simulink model "FreqSweep"  (Simulink 7.6)
settings: Solver=FixedStepDiscrete  SolverMode=SingleTasking  StartTime=0.0  StopTime=137*20*8*4  FixedStep=1  RelTol=1e-3
PreLoadFcn:
  | close all
  | clear all
  | FilterOrder = 32
  | InputBitWidth = 8
  | LowPassFreqBand = [0 0.01 0.2 1];
  | LowPassMagnBand = [1 0.9 0.0001 0.0001];
  | 
  | FlCoef = firls(FilterOrder,LowPassFreqBand,LowPassMagnBand);
  | 
  | CoefBitWidth = InputBitWidth + ceil(log2((max(abs(FlCoef))/min(abs(FlCoef)))))
  | 
  | ScalingFactor = (2^(CoefBitWidth-1))-1;
  | FpCoef = fix(ScalingFactor * FlCoef);
  | %plot(FpCoef,'o');
  | %title('Fixed-point scaled coefficient value');
  | ImpulseData = zeros(1,1000);
  | ImpulseData(1) = 100;
  | h = conv(ImpulseData,FpCoef);
  | %fftplot(h);
  | %title('FIR Frequency response');
  | FirSamplingPeriod=1;
  | 
  | cordic_precision=20;
  | ScalingFactor = (2^(cordic_precision-1))-1;
  | K=1.0;
  | for i=1:cordic_precision
  |   cordic_atan_table(i) = round(atan(K)*ScalingFactor);
  |   K=0.5*K;
  | end;
  | %disp(['cordic_precision =' num2str(cordic_precision)]);
  | %disp(['cordic_atan_table =' num2str(cordic_atan_table)]);
InitFcn:
  | %% DSPBuilder Start
  | alt_dspbuilder_update_model(bdroot)
  | %% DSPBuilder End
libraries: allblocks_alteradspbuilder2 x97, simulink x1
settings Model: Creator=akarapet  LastModifiedBy=akarapet
settings DataIOCC: SignalLoggingName=sigsOut
settings OptimizationCC: InlineInvariantSignals=on  InitFltsAndDblsToZero=on
settings DebuggingCC: SaveWithParameterizedLinksMsg=none  SignalResolutionControl=TryResolveAllWithWarning  SolverPrmCheckMsg=none  MultiTaskDSMMsg=warning  MultiTaskCondExecSysMsg=none  StrictBusMsg=None
settings HardwareCC: TargetUnknown=on
settings RTWCC: IncludeERTFirstTime=on
settings GRTTargetCC: TargetFcnLib=ansi_tfl_tmw.mat

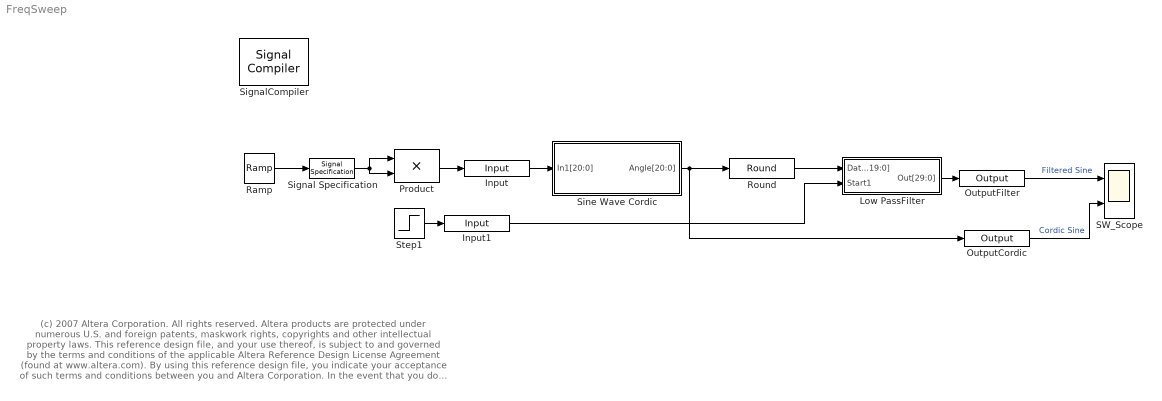
== system FreqSweep ==
  note: (c) 2007 Altera Corporation. All rights reserved.  Altera products are protected under numerous U.S. and foreign patents, maskwork rights, copyrights and other intellectual property laws.
      | This reference design file, and your use thereof, is subject to and governed by the terms and conditions of the applicable Altera Reference Design License Agreement (found at www.altera.com).
      | By using this reference design file, you indicate your acceptance of such terms and conditions between you and Altera Corporation.
      | In the event that you do not agree with such terms and conditions, you may not use the reference design file and please promptly destroy any copies you have made.
      | This reference design file being provided on an "as-is" basis and as an accommodation and therefore all warranties, representations or guarantees of any kind (whether express, implied or statutory)
      | including, without limitation, warranties of merchantability, non-infringement, or fitness for a particular purpose, are specifically disclaimed.
      | By making this reference design file available, Altera expressly does not recommend, suggest or require that this reference design file be used in combination with any other product not provided by Altera
  Input : allblocks_alteradspbuilder2/Input  iofile=/data/akarapet/qshell_linux64_test/p4/dsp_builder/dsp_builder2/Documentation/DesignExamples/Tutorials/HIL/FreqSweep/tb_FreqSweep/FreqSweep_Input.salt  BusType=Unsigned Integer  bwl=21  bwr=0  SpecifyClock=off  PORTTYPE=Input  externalType=Inferred  allowFloatingPointOverride=on  logOutputs=off
  Input1 : allblocks_alteradspbuilder2/Input  iofile=/data/akarapet/qshell_linux64_test/p4/dsp_builder/dsp_builder2/Documentation/DesignExamples/Tutorials/HIL/FreqSweep/tb_FreqSweep/FreqSweep_Input1.salt  BusType=Single Bit  bwl=1  bwr=0  SpecifyClock=off  PORTTYPE=Input  externalType=Inferred  allowFloatingPointOverride=on  logOutputs=off
  Low PassFilter : Subsystem  AncestorBlock=ALTELINK/AltLab/HDL SubSystem
      mask Type: SubSystem AlteraBlockSet
  OutputCordic : allblocks_alteradspbuilder2/Output  iofile=/data/akarapet/qshell_linux64_test/p4/dsp_builder/dsp_builder2/Documentation/DesignExamples/Tutorials/HIL/FreqSweep/tb_FreqSweep/FreqSweep_OutputCordic.capture  BusType=Signed Integer  bwl=21  bwr=0  externalType=Inferred  PORTTYPE=Output  allowFloatingPointOverride=on  logOutputs=off
  OutputFilter : allblocks_alteradspbuilder2/Output  iofile=/data/akarapet/qshell_linux64_test/p4/dsp_builder/dsp_builder2/Documentation/DesignExamples/Tutorials/HIL/FreqSweep/tb_FreqSweep/FreqSweep_OutputFilter.capture  BusType=Signed Integer  bwl=30  bwr=0  externalType=Inferred  PORTTYPE=Output  allowFloatingPointOverride=on  logOutputs=off
  Product : Product  SaturateOnIntegerOverflow=on  OutDataTypeStr=Inherit: Same as first input
  Ramp : simulink/Sources/Ramp  SystemSampleTime=-1  slope=.01  start=0  X0=0
  Round : allblocks_alteradspbuilder2/Round  BusType=Signed Integer  bwl=21  bwr=0  bitsToRemove=1  roundMode=ROUND_UP_SYM  userRoundMode=Round Away From Zero  pipeline=on  pipeline_display=1  use_ena=off  use_aclr=off
  SW_Scope : Scope  NumInputPorts=2
      settings: YMin=-1.1e+006~-550000  YMax=1.1e+006~550000  Decimation=20
  Signal Specification : SignalSpecification  SampleTime=1
  SignalCompiler : allblocks_alteradspbuilder2/Signal Compiler  DeviceFamily=Cyclone III  DeviceName=EP3C120F780C7  EnableSignalTap=off  SignalTapDepth=128  UseBoardBlock=off  StpUseDefaultClock=on  StpClock=Clock  ExportDir=/data/akarapet/qshell_linux64_test/p4/dsp_builder/dsp_builder2/Documentation/DesignExamples/Tutorials/HIL/FreqSweep/.
  Sine Wave Cordic : Subsystem
      mask Type: SubSystem AlteraBlockSet
  Step1 : Step  SampleTime=1
  wires:
  Ramp/1 -> Signal Specification/1
  Sine Wave Cordic/1(Angle[20:0]) -> OutputCordic/1, Round/1
  Input1/1 -> Low PassFilter/2(Start1)
  Step1/1 -> Input1/1
  Round/1 -> Low PassFilter/1(DataIn[19:0])
  Product/1 -> Input/1
  Input/1 -> Sine Wave Cordic/1(In1[20:0])
  Low PassFilter/1(Out[29:0]) -> OutputFilter/1
  Signal Specification/1 -> Product/1, Product/2
  OutputFilter/1 -> SW_Scope/1  "Filtered Sine"
  OutputCordic/1 -> SW_Scope/2  "Cordic Sine"

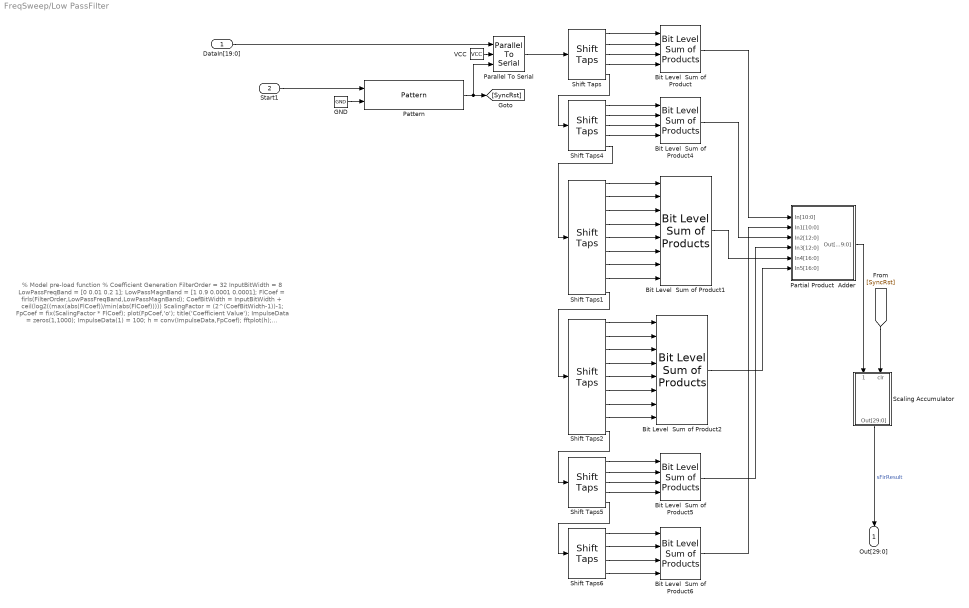
== system FreqSweep/Low PassFilter ==
  note: % Model pre-load function
      | % Coefficient Generation
      | FilterOrder = 32
      | InputBitWidth = 8
      | LowPassFreqBand = [0 0.01 0.2 1];
      | LowPassMagnBand = [1 0.9 0.0001 0.0001];
      |
      | FlCoef = firls(FilterOrder,LowPassFreqBand,LowPassMagnBand);
      |
      | CoefBitWidth = InputBitWidth + ceil(log2((max(abs(FlCoef))/min(abs(FlCoef)))))
      | ScalingFactor = (2^(CoefBitWidth-1))-1;
      |
      | FpCoef = fix(ScalingFactor * FlCoef);
      |
      | plot(FpCoef,'o');
      | title('Coefficient Value');
      | ImpulseData = zeros(1,1000);
      | ImpulseData(1) = 100;
      | h = conv(ImpulseData,FpCoef);
      | fftplot(h);
      | title('Frequency response');
      | FirSamplingPeriod=1;
  DataIn[19:0] : Inport
  Start1 : Inport  Port=2
  Bit Level  Sum of Product : allblocks_alteradspbuilder2/Bit Level Sum of Products  number_of_coefficients=4  BusType=Signed Integer  bwl=9  bwr=0  coefficients=[FpCoef(1:4)]  register_inputs=off  pipeline_display=0  use_ena=off  use_sclr=off  allowFloatingPointOverride=on  logOutputs=off  logFile=/data/akarapet/qshell_linux64_test/p4/dsp_builder/dsp_builder2/Documentation/DesignExamples/Tutorials/HIL/FreqSweep/tb_FreqSweep/FreqSweep_Low+PassFilter_Bit+Level+%0ASum+of+Product.fixedpointlog
  Bit Level  Sum of Product1 : allblocks_alteradspbuilder2/Bit Level Sum of Products  number_of_coefficients=8  BusType=Signed Integer  bwl=14  bwr=0  coefficients=[FpCoef(9:16)]  register_inputs=off  pipeline_display=0  use_ena=off  use_sclr=off  allowFloatingPointOverride=on  logOutputs=off  logFile=/data/akarapet/qshell_linux64_test/p4/dsp_builder/dsp_builder2/Documentation/DesignExamples/Tutorials/HIL/FreqSweep/tb_FreqSweep/FreqSweep_Low+PassFilter_Bit+Level+%0ASum+of+Product1.fixedpointlog
  Bit Level  Sum of Product2 : allblocks_alteradspbuilder2/Bit Level Sum of Products  number_of_coefficients=8  BusType=Signed Integer  bwl=14  bwr=0  coefficients=[FpCoef(17:24)]  register_inputs=off  pipeline_display=0  use_ena=off  use_sclr=off  allowFloatingPointOverride=on  logOutputs=off  logFile=/data/akarapet/qshell_linux64_test/p4/dsp_builder/dsp_builder2/Documentation/DesignExamples/Tutorials/HIL/FreqSweep/tb_FreqSweep/FreqSweep_Low+PassFilter_Bit+Level+%0ASum+of+Product2.fixedpointlog
  Bit Level  Sum of Product4 : allblocks_alteradspbuilder2/Bit Level Sum of Products  number_of_coefficients=4  BusType=Signed Integer  bwl=11  bwr=0  coefficients=[FpCoef(5:8)]  register_inputs=off  pipeline_display=0  use_ena=off  use_sclr=off  allowFloatingPointOverride=on  logOutputs=off  logFile=/data/akarapet/qshell_linux64_test/p4/dsp_builder/dsp_builder2/Documentation/DesignExamples/Tutorials/HIL/FreqSweep/tb_FreqSweep/FreqSweep_Low+PassFilter_Bit+Level+%0ASum+of+Product4.fixedpointlog
  Bit Level  Sum of Product5 : allblocks_alteradspbuilder2/Bit Level Sum of Products  number_of_coefficients=4  BusType=Signed Integer  bwl=11  bwr=0  coefficients=[FpCoef(25:28)]  register_inputs=off  pipeline_display=0  use_ena=off  use_sclr=off  allowFloatingPointOverride=on  logOutputs=off  logFile=/data/akarapet/qshell_linux64_test/p4/dsp_builder/dsp_builder2/Documentation/DesignExamples/Tutorials/HIL/FreqSweep/tb_FreqSweep/FreqSweep_Low+PassFilter_Bit+Level+%0ASum+of+Product5.fixedpointlog
  Bit Level  Sum of Product6 : allblocks_alteradspbuilder2/Bit Level Sum of Products  number_of_coefficients=4  BusType=Signed Integer  bwl=9  bwr=0  coefficients=[FpCoef(29:32)]  register_inputs=off  pipeline_display=0  use_ena=off  use_sclr=off  allowFloatingPointOverride=on  logOutputs=off  logFile=/data/akarapet/qshell_linux64_test/p4/dsp_builder/dsp_builder2/Documentation/DesignExamples/Tutorials/HIL/FreqSweep/tb_FreqSweep/FreqSweep_Low+PassFilter_Bit+Level+%0ASum+of+Product6.fixedpointlog
  GND : allblocks_alteradspbuilder2/GND  SpecifyClock=off
  Parallel To Serial : allblocks_alteradspbuilder2/Parallel To Serial  BusType=Signed Integer  bwl=20  bwr=0  msbfirsttext=LSB First  msbfirst=0  repeatlastbit=on  use_ena=on  use_sclr=off
  Partial Product  Adder : Subsystem  AncestorBlock=ALTELINK/AltLab/HDL SubSystem
      mask Type: SubSystem AlteraBlockSet
  Pattern : allblocks_alteradspbuilder2/Pattern  Sequence=10000000000000000000  SpecifyClock=off  use_ena=on  use_sclr=on
  Scaling Accumulator : Subsystem  AncestorBlock=ALTELINK/AltLab/HDL SubSystem
      mask Type: SubSystem AlteraBlockSet
  Shift Taps : allblocks_alteradspbuilder2/Shift Taps  number_of_taps=4  tap_distance=20  use_shiftout=on  use_ena=off  use_sclr=off  use_dedicated_circuitry=on  ram_type=AUTO  allowFloatingPointOverride=on  logOutputs=off  logFile=/data/akarapet/qshell_linux64_test/p4/dsp_builder/dsp_builder2/Documentation/DesignExamples/Tutorials/HIL/FreqSweep/tb_FreqSweep/FreqSweep_Low+PassFilter_Shift+Taps%3A%3At.fixedpointlog,/data/akarapet/qshell_linux64_test/p4/dsp_builder/dsp_builder2/Documentation/DesignExamples/Tutorials/HIL/FreqSweep/tb_FreqSweep/FreqSweep_Low+PassFilter_Shift+Taps%3A%3At.fixedpointlog,/data/akarapet/qshell_linux64_test/p4/dsp_builder/dsp_builder2/Documentation/DesignExamples/Tutorials/HIL/FreqSweep/tb_FreqSweep/FreqSweep_Low+PassFilter_Shift+Taps%3A%3At.fixedpointlog,/data/akarapet/qshell_linux64_test/p4/dsp_builder/dsp_builder2/Documentation/DesignExamples/Tutorials/HIL/FreqSweep/tb_FreqSweep/FreqSweep_Low+PassFilter_Shift+Taps%3A%3At.fixedpointlog,/data/akarapet/qshell_linux64_test/p4/dsp_builder/dsp_builder2/Documentation/DesignExamples/Tutorials/HIL/FreqSweep/tb_FreqSweep/FreqSweep_Low+PassFilter_Shift+Taps%3A%3Ashiftout.fixedpointlog,
  Shift Taps1 : allblocks_alteradspbuilder2/Shift Taps  number_of_taps=8  tap_distance=20  use_shiftout=on  use_ena=off  use_sclr=off  use_dedicated_circuitry=on  ram_type=AUTO  allowFloatingPointOverride=on  logOutputs=off  logFile=/data/akarapet/qshell_linux64_test/p4/dsp_builder/dsp_builder2/Documentation/DesignExamples/Tutorials/HIL/FreqSweep/tb_FreqSweep/FreqSweep_Low+PassFilter_Shift+Taps1%3A%3At.fixedpointlog,/data/akarapet/qshell_linux64_test/p4/dsp_builder/dsp_builder2/Documentation/DesignExamples/Tutorials/HIL/FreqSweep/tb_FreqSweep/FreqSweep_Low+PassFilter_Shift+Taps1%3A%3At.fixedpointlog,/data/akarapet/qshell_linux64_test/p4/dsp_builder/dsp_builder2/Documentation/DesignExamples/Tutorials/HIL/FreqSweep/tb_FreqSweep/FreqSweep_Low+PassFilter_Shift+Taps1%3A%3At.fixedpointlog,/data/akarapet/qshell_linux64_test/p4/dsp_builder/dsp_builder2/Documentation/DesignExamples/Tutorials/HIL/FreqSweep/tb_FreqSweep/FreqSweep_Low+PassFilter_Shift+Taps1%3A%3At.fixedpointlog,/data/akarapet/qshell_linux64_test/p4/dsp_builder/dsp_builder2/Documentation/DesignExamples/Tutorials/HIL/FreqSweep/tb_FreqSweep/FreqSweep_Low+PassFilter_Shift+Taps1%3A%3At.fixedpointlog,/data/akarapet/qshell_linux64_test/p4/dsp_builder/dsp_builder2/Documentation/DesignExamples/Tutorials/HIL/FreqSweep/tb_FreqSweep/FreqSweep_Low+PassFilter_Shift+Taps1%3A%3At.fixedpointlog,/data/akarapet/qshell_linux64_test/p4/dsp_builder/dsp_builder2/Documentation/DesignExamples/Tutorials/HIL/FreqSweep/tb_FreqSweep/FreqSweep_Low+PassFilter_Shift+Taps1%3A%3At.fixedpointlog,/data/akarapet/qshell_linux64_test/p4/dsp_builder/dsp_builder2/Documentation/DesignExamples/Tutorials/HIL/FreqSweep/tb_FreqSweep/FreqSweep_Low+PassFilter_Shift+Taps1%3A%3At.fixedpointlog,/data/akarapet/qshell_linux64_test/p4/dsp_builder/dsp_builder2/Documentation/DesignExamples/Tutorials/HIL/FreqSweep/tb_FreqSweep/FreqSweep_Low+PassFilter_Shift+Taps1%3A%3Ashiftout.fixedpointlog,
  Shift Taps2 : allblocks_alteradspbuilder2/Shift Taps  number_of_taps=8  tap_distance=20  use_shiftout=on  use_ena=off  use_sclr=off  use_dedicated_circuitry=on  ram_type=AUTO  allowFloatingPointOverride=on  logOutputs=off  logFile=/data/akarapet/qshell_linux64_test/p4/dsp_builder/dsp_builder2/Documentation/DesignExamples/Tutorials/HIL/FreqSweep/tb_FreqSweep/FreqSweep_Low+PassFilter_Shift+Taps2%3A%3At.fixedpointlog,/data/akarapet/qshell_linux64_test/p4/dsp_builder/dsp_builder2/Documentation/DesignExamples/Tutorials/HIL/FreqSweep/tb_FreqSweep/FreqSweep_Low+PassFilter_Shift+Taps2%3A%3At.fixedpointlog,/data/akarapet/qshell_linux64_test/p4/dsp_builder/dsp_builder2/Documentation/DesignExamples/Tutorials/HIL/FreqSweep/tb_FreqSweep/FreqSweep_Low+PassFilter_Shift+Taps2%3A%3At.fixedpointlog,/data/akarapet/qshell_linux64_test/p4/dsp_builder/dsp_builder2/Documentation/DesignExamples/Tutorials/HIL/FreqSweep/tb_FreqSweep/FreqSweep_Low+PassFilter_Shift+Taps2%3A%3At.fixedpointlog,/data/akarapet/qshell_linux64_test/p4/dsp_builder/dsp_builder2/Documentation/DesignExamples/Tutorials/HIL/FreqSweep/tb_FreqSweep/FreqSweep_Low+PassFilter_Shift+Taps2%3A%3At.fixedpointlog,/data/akarapet/qshell_linux64_test/p4/dsp_builder/dsp_builder2/Documentation/DesignExamples/Tutorials/HIL/FreqSweep/tb_FreqSweep/FreqSweep_Low+PassFilter_Shift+Taps2%3A%3At.fixedpointlog,/data/akarapet/qshell_linux64_test/p4/dsp_builder/dsp_builder2/Documentation/DesignExamples/Tutorials/HIL/FreqSweep/tb_FreqSweep/FreqSweep_Low+PassFilter_Shift+Taps2%3A%3At.fixedpointlog,/data/akarapet/qshell_linux64_test/p4/dsp_builder/dsp_builder2/Documentation/DesignExamples/Tutorials/HIL/FreqSweep/tb_FreqSweep/FreqSweep_Low+PassFilter_Shift+Taps2%3A%3At.fixedpointlog,/data/akarapet/qshell_linux64_test/p4/dsp_builder/dsp_builder2/Documentation/DesignExamples/Tutorials/HIL/FreqSweep/tb_FreqSweep/FreqSweep_Low+PassFilter_Shift+Taps2%3A%3Ashiftout.fixedpointlog,
  Shift Taps4 : allblocks_alteradspbuilder2/Shift Taps  number_of_taps=4  tap_distance=20  use_shiftout=on  use_ena=off  use_sclr=off  use_dedicated_circuitry=on  ram_type=AUTO  allowFloatingPointOverride=on  logOutputs=off  logFile=/data/akarapet/qshell_linux64_test/p4/dsp_builder/dsp_builder2/Documentation/DesignExamples/Tutorials/HIL/FreqSweep/tb_FreqSweep/FreqSweep_Low+PassFilter_Shift+Taps4%3A%3At.fixedpointlog,/data/akarapet/qshell_linux64_test/p4/dsp_builder/dsp_builder2/Documentation/DesignExamples/Tutorials/HIL/FreqSweep/tb_FreqSweep/FreqSweep_Low+PassFilter_Shift+Taps4%3A%3At.fixedpointlog,/data/akarapet/qshell_linux64_test/p4/dsp_builder/dsp_builder2/Documentation/DesignExamples/Tutorials/HIL/FreqSweep/tb_FreqSweep/FreqSweep_Low+PassFilter_Shift+Taps4%3A%3At.fixedpointlog,/data/akarapet/qshell_linux64_test/p4/dsp_builder/dsp_builder2/Documentation/DesignExamples/Tutorials/HIL/FreqSweep/tb_FreqSweep/FreqSweep_Low+PassFilter_Shift+Taps4%3A%3At.fixedpointlog,/data/akarapet/qshell_linux64_test/p4/dsp_builder/dsp_builder2/Documentation/DesignExamples/Tutorials/HIL/FreqSweep/tb_FreqSweep/FreqSweep_Low+PassFilter_Shift+Taps4%3A%3Ashiftout.fixedpointlog,
  Shift Taps5 : allblocks_alteradspbuilder2/Shift Taps  number_of_taps=4  tap_distance=20  use_shiftout=on  use_ena=off  use_sclr=off  use_dedicated_circuitry=on  ram_type=AUTO  allowFloatingPointOverride=on  logOutputs=off  logFile=/data/akarapet/qshell_linux64_test/p4/dsp_builder/dsp_builder2/Documentation/DesignExamples/Tutorials/HIL/FreqSweep/tb_FreqSweep/FreqSweep_Low+PassFilter_Shift+Taps5%3A%3At.fixedpointlog,/data/akarapet/qshell_linux64_test/p4/dsp_builder/dsp_builder2/Documentation/DesignExamples/Tutorials/HIL/FreqSweep/tb_FreqSweep/FreqSweep_Low+PassFilter_Shift+Taps5%3A%3At.fixedpointlog,/data/akarapet/qshell_linux64_test/p4/dsp_builder/dsp_builder2/Documentation/DesignExamples/Tutorials/HIL/FreqSweep/tb_FreqSweep/FreqSweep_Low+PassFilter_Shift+Taps5%3A%3At.fixedpointlog,/data/akarapet/qshell_linux64_test/p4/dsp_builder/dsp_builder2/Documentation/DesignExamples/Tutorials/HIL/FreqSweep/tb_FreqSweep/FreqSweep_Low+PassFilter_Shift+Taps5%3A%3At.fixedpointlog,/data/akarapet/qshell_linux64_test/p4/dsp_builder/dsp_builder2/Documentation/DesignExamples/Tutorials/HIL/FreqSweep/tb_FreqSweep/FreqSweep_Low+PassFilter_Shift+Taps5%3A%3Ashiftout.fixedpointlog,
  Shift Taps6 : allblocks_alteradspbuilder2/Shift Taps  number_of_taps=4  tap_distance=20  use_shiftout=off  use_ena=off  use_sclr=off  use_dedicated_circuitry=on  ram_type=AUTO  allowFloatingPointOverride=on  logOutputs=off  logFile=/data/akarapet/qshell_linux64_test/p4/dsp_builder/dsp_builder2/Documentation/DesignExamples/Tutorials/HIL/FreqSweep/tb_FreqSweep/FreqSweep_Low+PassFilter_Shift+Taps6%3A%3At.fixedpointlog,/data/akarapet/qshell_linux64_test/p4/dsp_builder/dsp_builder2/Documentation/DesignExamples/Tutorials/HIL/FreqSweep/tb_FreqSweep/FreqSweep_Low+PassFilter_Shift+Taps6%3A%3At.fixedpointlog,/data/akarapet/qshell_linux64_test/p4/dsp_builder/dsp_builder2/Documentation/DesignExamples/Tutorials/HIL/FreqSweep/tb_FreqSweep/FreqSweep_Low+PassFilter_Shift+Taps6%3A%3At.fixedpointlog,/data/akarapet/qshell_linux64_test/p4/dsp_builder/dsp_builder2/Documentation/DesignExamples/Tutorials/HIL/FreqSweep/tb_FreqSweep/FreqSweep_Low+PassFilter_Shift+Taps6%3A%3At.fixedpointlog,
  VCC : allblocks_alteradspbuilder2/VCC  SpecifyClock=off
  Out[29:0] : Outport
  wires:
  DataIn[19:0]/1 -> Parallel To Serial/1
  Shift Taps1/1 -> Bit Level  Sum of Product1/1
  Shift Taps1/2 -> Bit Level  Sum of Product1/2
  Shift Taps1/3 -> Bit Level  Sum of Product1/3
  Shift Taps1/4 -> Bit Level  Sum of Product1/4
  Shift Taps1/5 -> Bit Level  Sum of Product1/5
  Shift Taps1/6 -> Bit Level  Sum of Product1/6
  Shift Taps1/7 -> Bit Level  Sum of Product1/7
  Shift Taps1/8 -> Bit Level  Sum of Product1/8
  Shift Taps2/1 -> Bit Level  Sum of Product2/1
  Shift Taps2/2 -> Bit Level  Sum of Product2/2
  Shift Taps2/3 -> Bit Level  Sum of Product2/3
  Shift Taps2/4 -> Bit Level  Sum of Product2/4
  Shift Taps2/5 -> Bit Level  Sum of Product2/5
  Shift Taps2/6 -> Bit Level  Sum of Product2/6
  Shift Taps2/7 -> Bit Level  Sum of Product2/7
  Shift Taps2/8 -> Bit Level  Sum of Product2/8
  Shift Taps1/9 -> Shift Taps2/1
  Parallel To Serial/1 -> Shift Taps/1
  Pattern/1 -> [SyncRst], Parallel To Serial/3
  GND/1 -> Pattern/2
  [SyncRst] -> Scaling Accumulator/2(clr)
  Shift Taps/1 -> Bit Level  Sum of Product/1
  Shift Taps/2 -> Bit Level  Sum of Product/2
  Shift Taps/3 -> Bit Level  Sum of Product/3
  Shift Taps/4 -> Bit Level  Sum of Product/4
  Shift Taps4/1 -> Bit Level  Sum of Product4/1
  Shift Taps4/2 -> Bit Level  Sum of Product4/2
  Shift Taps4/3 -> Bit Level  Sum of Product4/3
  Shift Taps4/4 -> Bit Level  Sum of Product4/4
  Shift Taps/5 -> Shift Taps4/1
  Shift Taps4/5 -> Shift Taps1/1
  Shift Taps5/1 -> Bit Level  Sum of Product5/1
  Shift Taps5/2 -> Bit Level  Sum of Product5/2
  Shift Taps5/3 -> Bit Level  Sum of Product5/3
  Shift Taps5/4 -> Bit Level  Sum of Product5/4
  Shift Taps6/1 -> Bit Level  Sum of Product6/1
  Shift Taps6/2 -> Bit Level  Sum of Product6/2
  Shift Taps6/3 -> Bit Level  Sum of Product6/3
  Shift Taps6/4 -> Bit Level  Sum of Product6/4
  Shift Taps5/5 -> Shift Taps6/1
  Shift Taps2/9 -> Shift Taps5/1
  Bit Level  Sum of Product5/1 -> Partial Product  Adder/4(In3[12:0])
  Bit Level  Sum of Product/1 -> Partial Product  Adder/1(In[10:0])
  Bit Level  Sum of Product6/1 -> Partial Product  Adder/2(In1[10:0])
  Bit Level  Sum of Product4/1 -> Partial Product  Adder/3(In2[12:0])
  Bit Level  Sum of Product1/1 -> Partial Product  Adder/5(In4[16:0])
  Bit Level  Sum of Product2/1 -> Partial Product  Adder/6(In5[16:0])
  VCC/1 -> Parallel To Serial/2
  Scaling Accumulator/1(Out[29:0]) -> Out[29:0]/1  "sFirResult"
  Start1/1 -> Pattern/1
  Partial Product  Adder/1(Out[19:0]) -> Scaling Accumulator/1(In[19:0])

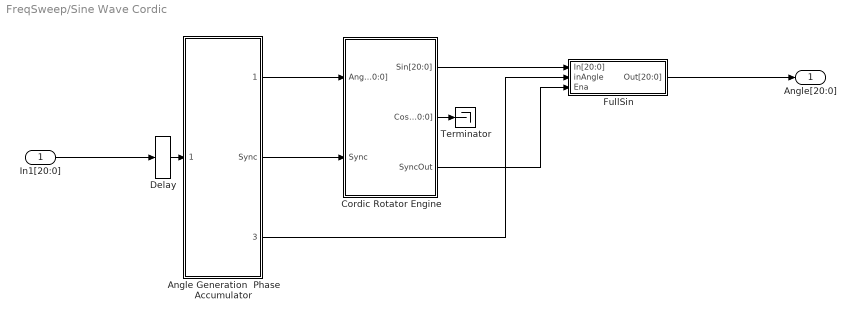
== system FreqSweep/Sine Wave Cordic ==
  In1[20:0] : Inport
  Angle Generation  Phase Accumulator : Subsystem  AncestorBlock=ALTELINK/AltLab/HDL SubSystem
      mask Type: SubSystem AlteraBlockSet
  Cordic Rotator Engine : Subsystem  AncestorBlock=ALTELINK/AltLab/HDL SubSystem
      mask Type: SubSystem AlteraBlockSet
  Delay : allblocks_alteradspbuilder2/Delay  pipeline=1  pipeline_display=1  ClockPhase=1  use_ena=off  use_sclr=off  allowFloatingPointOverride=on  logOutputs=off  logFile=/data/akarapet/qshell_linux64_test/p4/dsp_builder/dsp_builder2/Documentation/DesignExamples/Tutorials/HIL/FreqSweep/tb_FreqSweep/FreqSweep_Sine+Wave+Cordic_Delay.fixedpointlog  use_init=off  reset_value=1
  FullSin : Subsystem  AncestorBlock=ALTELINK/AltLab/HDL SubSystem
      mask Type: SubSystem AlteraBlockSet
  Terminator : Terminator
  Angle[20:0] : Outport
  wires:
  Cordic Rotator Engine/3(SyncOut) -> FullSin/3(Ena)
  Angle Generation  Phase Accumulator/2(Sync) -> Cordic Rotator Engine/2(Sync)
  Angle Generation  Phase Accumulator/1(Angle[20:0]) -> Cordic Rotator Engine/1(Angle[20:0])
  Angle Generation  Phase Accumulator/3(oNegAngle) -> FullSin/2(inAngle)
  Cordic Rotator Engine/1(Sin[20:0]) -> FullSin/1(In[20:0])
  In1[20:0]/1 -> Delay/1
  Delay/1 -> Angle Generation  Phase Accumulator/1(In1[20:0])
  Cordic Rotator Engine/2(Cos[20:0]) -> Terminator/1
  FullSin/1(Out[20:0]) -> Angle[20:0]/1

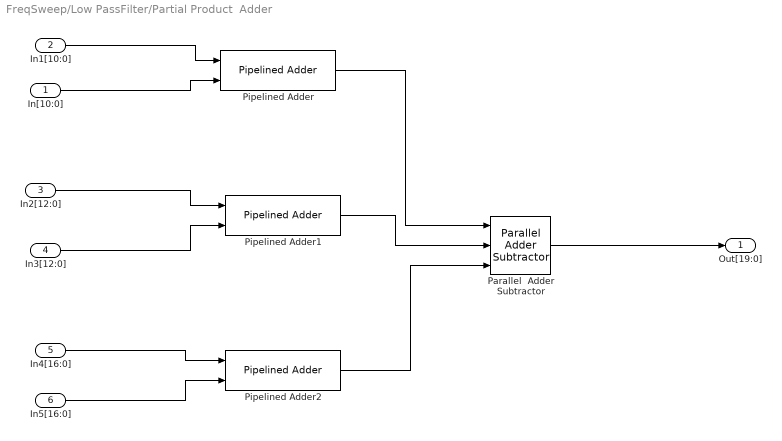
== system FreqSweep/Low PassFilter/Partial Product  Adder ==
  In[10:0] : Inport
  In1[10:0] : Inport  Port=2
  In2[12:0] : Inport  Port=3
  In3[12:0] : Inport  Port=4
  In4[16:0] : Inport  Port=5
  In5[16:0] : Inport  Port=6
  Parallel  Adder Subtractor : allblocks_alteradspbuilder2/Parallel Adder Subtractor  number_of_inputs=3  direction=++  use_pipeline=on  pipeline_display=2  phase_selection=1  use_ena=off  use_aclr=off  allowFloatingPointOverride=on  logOutputs=off  logFile=/data/akarapet/qshell_linux64_test/p4/dsp_builder/dsp_builder2/Documentation/DesignExamples/Tutorials/HIL/FreqSweep/tb_FreqSweep/FreqSweep_Low+PassFilter_Partial+Product+%0AAdder_Parallel+%0AAdder+Subtractor.fixedpointlog
  Pipelined Adder : allblocks_alteradspbuilder2/Pipelined Adder  BusType=Signed Integer  bwl=12  bwr=0  pipeline=2  pipeline_display=2  AddSubDirection=ADD  use_cin=off  use_ovl=off  use_addsub=off  use_ena=off  use_aclr=off  or_aclr_inputs=on
  Pipelined Adder1 : allblocks_alteradspbuilder2/Pipelined Adder  BusType=Signed Integer  bwl=14  bwr=0  pipeline=2  pipeline_display=2  AddSubDirection=ADD  use_cin=off  use_ovl=off  use_addsub=off  use_ena=off  use_aclr=off  or_aclr_inputs=on
  Pipelined Adder2 : allblocks_alteradspbuilder2/Pipelined Adder  BusType=Signed Integer  bwl=18  bwr=0  pipeline=2  pipeline_display=2  AddSubDirection=ADD  use_cin=off  use_ovl=off  use_addsub=off  use_ena=off  use_aclr=off  or_aclr_inputs=on
  Out[19:0] : Outport
  wires:
  In[10:0]/1 -> Pipelined Adder/2
  In1[10:0]/1 -> Pipelined Adder/1
  In2[12:0]/1 -> Pipelined Adder1/1
  In3[12:0]/1 -> Pipelined Adder1/2
  In4[16:0]/1 -> Pipelined Adder2/1
  In5[16:0]/1 -> Pipelined Adder2/2
  Pipelined Adder/1 -> Parallel  Adder Subtractor/1
  Pipelined Adder1/1 -> Parallel  Adder Subtractor/2
  Pipelined Adder2/1 -> Parallel  Adder Subtractor/3
  Parallel  Adder Subtractor/1 -> Out[19:0]/1

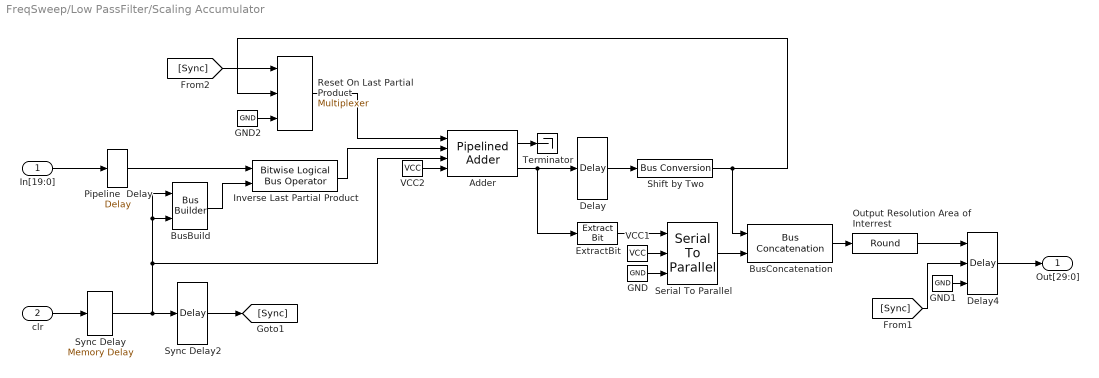
== system FreqSweep/Low PassFilter/Scaling Accumulator ==
  In[19:0] : Inport
  clr : Inport  Port=2
  Adder : allblocks_alteradspbuilder2/Pipelined Adder  BusType=Signed Integer  bwl=21  bwr=0  pipeline=0  pipeline_display=0  AddSubDirection=ADD  use_cin=on  use_ovl=on  use_addsub=on  use_ena=on  use_aclr=on  or_aclr_inputs=on
  BusBuild : allblocks_alteradspbuilder2/Bus Builder  BusType=Signed Integer  bwl=2  bwr=0  pipeline_display=0
  BusConcatenation : allblocks_alteradspbuilder2/Bus Concatenation  isSigned=on  awidth=20  bwidth=20  pipeline_display=0
  Delay : allblocks_alteradspbuilder2/Delay  pipeline=1  pipeline_display=1  ClockPhase=1  use_ena=off  use_sclr=off  allowFloatingPointOverride=on  logOutputs=off  logFile=/data/akarapet/qshell_linux64_test/p4/dsp_builder/dsp_builder2/Documentation/DesignExamples/Tutorials/HIL/FreqSweep/tb_FreqSweep/FreqSweep_Low+PassFilter_Scaling+Accumulator_Delay.fixedpointlog  use_init=off  reset_value=1
  Delay4 : allblocks_alteradspbuilder2/Delay  pipeline=1  pipeline_display=1  ClockPhase=1  use_ena=on  use_sclr=on  allowFloatingPointOverride=on  logOutputs=off  logFile=/data/akarapet/qshell_linux64_test/p4/dsp_builder/dsp_builder2/Documentation/DesignExamples/Tutorials/HIL/FreqSweep/tb_FreqSweep/FreqSweep_Low+PassFilter_Scaling+Accumulator_Delay4.fixedpointlog  use_init=off  reset_value=1
  ExtractBit : allblocks_alteradspbuilder2/Extract Bit  BusType=Signed Fractional  bwl=21  bwr=0  bitToSelect=0  pipeline_display=0
  GND : allblocks_alteradspbuilder2/GND  SpecifyClock=off
  GND1 : allblocks_alteradspbuilder2/GND  SpecifyClock=off
  GND2 : allblocks_alteradspbuilder2/GND  SpecifyClock=off
  Inverse Last Partial Product : allblocks_alteradspbuilder2/Bitwise Logical Bus Operator  BusType=Signed Integer  bwl=20  bwr=0  LogicalOperator=XOR  pipeline_display=0
  Output Resolution Area of Interrest : allblocks_alteradspbuilder2/Round  BusType=Signed Integer  bwl=40  bwr=0  bitsToRemove=10  roundMode=ROUND_UP_SYM  userRoundMode=Round Away From Zero  pipeline=off  pipeline_display=0  use_ena=off  use_aclr=off
  Pipeline  Delay : allblocks_alteradspbuilder2/Delay  pipeline=1  pipeline_display=1  ClockPhase=1  use_ena=off  use_sclr=off  allowFloatingPointOverride=on  logOutputs=off  logFile=/data/akarapet/qshell_linux64_test/p4/dsp_builder/dsp_builder2/Documentation/DesignExamples/Tutorials/HIL/FreqSweep/tb_FreqSweep/FreqSweep_Low+PassFilter_Scaling+Accumulator_Pipeline+%0ADelay.fixedpointlog  use_init=off  reset_value=1
  Reset On Last Partial Product : allblocks_alteradspbuilder2/Multiplexer  numInputs=2  pipeline=0  oneHot=off  pipeline_display=0  use_ena=off  use_aclr=off  allowFloatingPointOverride=on  logOutputs=off  logFile=/data/akarapet/qshell_linux64_test/p4/dsp_builder/dsp_builder2/Documentation/DesignExamples/Tutorials/HIL/FreqSweep/tb_FreqSweep/FreqSweep_Low+PassFilter_Scaling+Accumulator_Reset+On%0ALast+Partial+Product.fixedpointlog
  Serial To Parallel : allblocks_alteradspbuilder2/Serial To Parallel  BusType=Unsigned Integer  bwl=20  bwr=0  msbfirsttext=LSB First  msbfirst=0  use_ena=on  use_sclr=on
  Shift by Two : allblocks_alteradspbuilder2/Bus Conversion  BusType=Signed Integer  ibwl=21  ibwr=0  bwl=20  bwr=0  bitToConnectToOutputLSB=1  round=off  saturate=off  pipeline_display=0
  Sync Delay : allblocks_alteradspbuilder2/Memory Delay  BusType=Inferred  bwl=8  bwr=0  pipeline=5  pipeline_display=5  ram_type=AUTO  use_ena=off  use_sclr=off  allowFloatingPointOverride=on  logOutputs=off  logFile=/data/akarapet/qshell_linux64_test/p4/dsp_builder/dsp_builder2/Documentation/DesignExamples/Tutorials/HIL/FreqSweep/tb_FreqSweep/FreqSweep_Low+PassFilter_Scaling+Accumulator_Sync+Delay.fixedpointlog
  Sync Delay2 : allblocks_alteradspbuilder2/Delay  pipeline=1  pipeline_display=1  ClockPhase=1  use_ena=off  use_sclr=off  allowFloatingPointOverride=on  logOutputs=off  logFile=/data/akarapet/qshell_linux64_test/p4/dsp_builder/dsp_builder2/Documentation/DesignExamples/Tutorials/HIL/FreqSweep/tb_FreqSweep/FreqSweep_Low+PassFilter_Scaling+Accumulator_Sync+Delay2.fixedpointlog  use_init=off  reset_value=1
  Terminator : Terminator
  VCC1 : allblocks_alteradspbuilder2/VCC  SpecifyClock=off
  VCC2 : allblocks_alteradspbuilder2/VCC  SpecifyClock=off
  Out[29:0] : Outport
  wires:
  clr/1 -> Sync Delay/1
  In[19:0]/1 -> Pipeline  Delay/1
  Delay/1 -> Shift by Two/1
  Shift by Two/1 -> BusConcatenation/1, Reset On Last Partial Product/2
  VCC1/1 -> Serial To Parallel/2
  GND/1 -> Serial To Parallel/3
  Delay4/1 -> Out[29:0]/1
  GND1/1 -> Delay4/3
  ExtractBit/1 -> Serial To Parallel/1
  Reset On Last Partial Product/1 -> Adder/1
  GND2/1 -> Reset On Last Partial Product/3
  [Sync] -> Delay4/2
  [Sync] -> Reset On Last Partial Product/1
  VCC2/1 -> Adder/4
  Adder/2 -> Delay/1, ExtractBit/1
  Sync Delay/1 -> Sync Delay2/1, BusBuild/2, BusBuild/1, Adder/3
  Inverse Last Partial Product/1 -> Adder/2
  Pipeline  Delay/1 -> Inverse Last Partial Product/1
  Sync Delay2/1 -> [Sync]
  BusBuild/1 -> Inverse Last Partial Product/2
  Adder/1 -> Terminator/1
  Serial To Parallel/1 -> BusConcatenation/2
  BusConcatenation/1 -> Output Resolution Area of Interrest/1
  Output Resolution Area of Interrest/1 -> Delay4/1

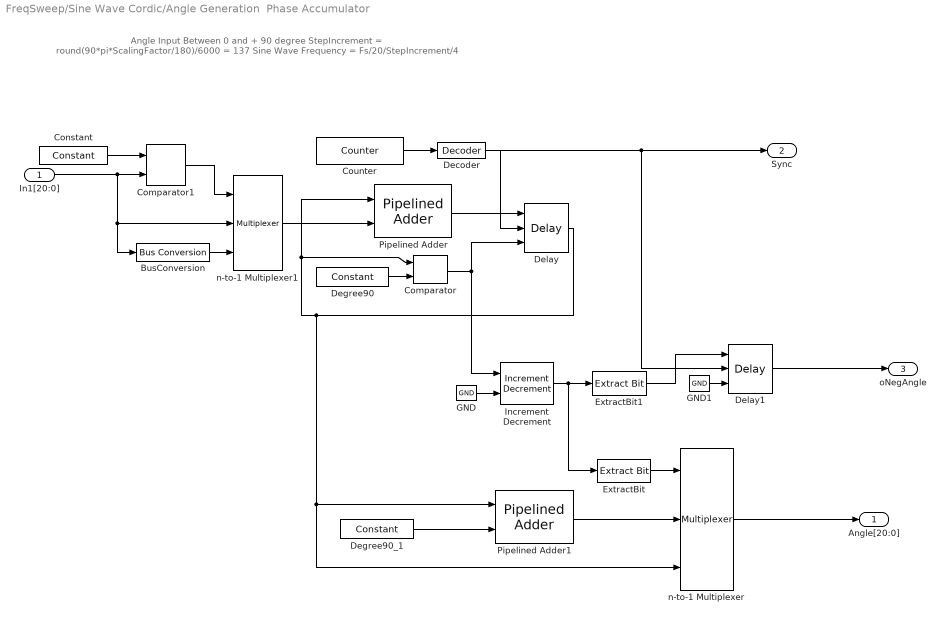
== system FreqSweep/Sine Wave Cordic/Angle Generation  Phase Accumulator ==
  note: Angle Input Between 0 and + 90 degree
      | StepIncrement = round(90*pi*ScalingFactor/180)/6000 = 137
      | Sine Wave Frequency = Fs/20/StepIncrement/4
  In1[20:0] : Inport
  BusConversion : allblocks_alteradspbuilder2/Bus Conversion  BusType=Unsigned Integer  ibwl=21  ibwr=0  bwl=17  bwr=0  bitToConnectToOutputLSB=0  round=off  saturate=off  pipeline_display=0
  Comparator : allblocks_alteradspbuilder2/Comparator  direction=a > b  pipeline_display=0  allowFloatingPointOverride=on  logOutputs=off  logFile=/data/akarapet/qshell_linux64_test/p4/dsp_builder/dsp_builder2/Documentation/DesignExamples/Tutorials/HIL/FreqSweep/tb_FreqSweep/FreqSweep_Sine+Wave+Cordic_Angle+Generation+%0APhase+Accumulator_Comparator.fixedpointlog
  Comparator1 : allblocks_alteradspbuilder2/Comparator  direction=a < b  pipeline_display=0  allowFloatingPointOverride=on  logOutputs=off  logFile=/data/akarapet/qshell_linux64_test/p4/dsp_builder/dsp_builder2/Documentation/DesignExamples/Tutorials/HIL/FreqSweep/tb_FreqSweep/FreqSweep_Sine+Wave+Cordic_Angle+Generation+%0APhase+Accumulator_Comparator1.fixedpointlog
  Constant : allblocks_alteradspbuilder2/Constant  mask_cst=2^17-+2^16  BusType=Signed Integer  bwl=21  bwr=0  roundMode=Truncate  satMode=Wrap  SpecifyClock=off  allowFloatingPointOverride=on  logOutputs=off  logFile=/data/akarapet/qshell_linux64_test/p4/dsp_builder/dsp_builder2/Documentation/DesignExamples/Tutorials/HIL/FreqSweep/tb_FreqSweep/FreqSweep_Sine+Wave+Cordic_Angle+Generation+%0APhase+Accumulator_Constant.fixedpointlog
  Counter : allblocks_alteradspbuilder2/Counter  BusType=Unsigned Integer  bwl=5  bwr=0  use_modulo=on  modulo=20  SpecifyClock=off  direction=Increment  use_sload=off  use_sset=off  svalue=1  use_clk_ena=off  use_ena=off  use_sclr=off  pipeline_display=1
  Decoder : allblocks_alteradspbuilder2/Decoder  BusType=Unsigned Integer  bwl=5  bwr=0  registered=off  pipeline_display=0  value=0
  Degree90 : allblocks_alteradspbuilder2/Constant  mask_cst=round(90*pi*ScalingFactor/180)  BusType=Signed Integer  bwl=21  bwr=0  roundMode=Truncate  satMode=Wrap  SpecifyClock=off  allowFloatingPointOverride=on  logOutputs=off  logFile=/data/akarapet/qshell_linux64_test/p4/dsp_builder/dsp_builder2/Documentation/DesignExamples/Tutorials/HIL/FreqSweep/tb_FreqSweep/FreqSweep_Sine+Wave+Cordic_Angle+Generation+%0APhase+Accumulator_Degree90.fixedpointlog
  Degree90_1 : allblocks_alteradspbuilder2/Constant  mask_cst=round(90*pi*ScalingFactor/180)  BusType=Signed Integer  bwl=21  bwr=0  roundMode=Truncate  satMode=Wrap  SpecifyClock=off  allowFloatingPointOverride=on  logOutputs=off  logFile=/data/akarapet/qshell_linux64_test/p4/dsp_builder/dsp_builder2/Documentation/DesignExamples/Tutorials/HIL/FreqSweep/tb_FreqSweep/FreqSweep_Sine+Wave+Cordic_Angle+Generation+%0APhase+Accumulator_Degree90%5F1.fixedpointlog
  Delay : allblocks_alteradspbuilder2/Delay  pipeline=1  pipeline_display=1  ClockPhase=1  use_ena=on  use_sclr=on  allowFloatingPointOverride=on  logOutputs=off  logFile=/data/akarapet/qshell_linux64_test/p4/dsp_builder/dsp_builder2/Documentation/DesignExamples/Tutorials/HIL/FreqSweep/tb_FreqSweep/FreqSweep_Sine+Wave+Cordic_Angle+Generation+%0APhase+Accumulator_Delay.fixedpointlog  use_init=off  reset_value=1
  Delay1 : allblocks_alteradspbuilder2/Delay  pipeline=2  pipeline_display=2  ClockPhase=1  use_ena=on  use_sclr=on  allowFloatingPointOverride=on  logOutputs=off  logFile=/data/akarapet/qshell_linux64_test/p4/dsp_builder/dsp_builder2/Documentation/DesignExamples/Tutorials/HIL/FreqSweep/tb_FreqSweep/FreqSweep_Sine+Wave+Cordic_Angle+Generation+%0APhase+Accumulator_Delay1.fixedpointlog  use_init=off  reset_value=1
  ExtractBit : allblocks_alteradspbuilder2/Extract Bit  BusType=Signed Fractional  bwl=2  bwr=0  bitToSelect=0  pipeline_display=0
  ExtractBit1 : allblocks_alteradspbuilder2/Extract Bit  BusType=Signed Fractional  bwl=2  bwr=0  bitToSelect=1  pipeline_display=0
  GND : allblocks_alteradspbuilder2/GND  SpecifyClock=off
  GND1 : allblocks_alteradspbuilder2/GND  SpecifyClock=off
  Increment Decrement : allblocks_alteradspbuilder2/Increment Decrement  BusType=Unsigned Integer  bwl=2  bwr=0  SpecifyClock=off  clr_value=0  direction=Increment  phase_selection=1  use_ena=on  use_sclr=on  pipeline_display=1
  Pipelined Adder : allblocks_alteradspbuilder2/Pipelined Adder  BusType=Signed Integer  bwl=21  bwr=0  pipeline=0  pipeline_display=0  AddSubDirection=ADD  use_cin=off  use_ovl=off  use_addsub=off  use_ena=off  use_aclr=off  or_aclr_inputs=on
  Pipelined Adder1 : allblocks_alteradspbuilder2/Pipelined Adder  BusType=Signed Integer  bwl=21  bwr=0  pipeline=0  pipeline_display=0  AddSubDirection=SUB  use_cin=off  use_ovl=off  use_addsub=off  use_ena=off  use_aclr=off  or_aclr_inputs=on
  n-to-1 Multiplexer : allblocks_alteradspbuilder2/Multiplexer  numInputs=2  pipeline=0  oneHot=off  pipeline_display=0  use_ena=off  use_aclr=off  allowFloatingPointOverride=on  logOutputs=off  logFile=/data/akarapet/qshell_linux64_test/p4/dsp_builder/dsp_builder2/Documentation/DesignExamples/Tutorials/HIL/FreqSweep/tb_FreqSweep/FreqSweep_Sine+Wave+Cordic_Angle+Generation+%0APhase+Accumulator_n-to-1+Multiplexer.fixedpointlog
  n-to-1 Multiplexer1 : allblocks_alteradspbuilder2/Multiplexer  numInputs=2  pipeline=0  oneHot=off  pipeline_display=0  use_ena=off  use_aclr=off  allowFloatingPointOverride=on  logOutputs=off  logFile=/data/akarapet/qshell_linux64_test/p4/dsp_builder/dsp_builder2/Documentation/DesignExamples/Tutorials/HIL/FreqSweep/tb_FreqSweep/FreqSweep_Sine+Wave+Cordic_Angle+Generation+%0APhase+Accumulator_n-to-1+Multiplexer1.fixedpointlog
  Angle[20:0] : Outport
  Sync : Outport  Port=2
  oNegAngle : Outport  Port=3
  wires:
  Counter/1 -> Decoder/1
  Decoder/1 -> Delay/2, Delay1/2, Sync/1
  Pipelined Adder/1 -> Delay/1
  Delay/1 -> Comparator/1, Pipelined Adder/1, n-to-1 Multiplexer/3, Pipelined Adder1/1
  Comparator/1 -> Delay/3, Increment Decrement/1
  Degree90/1 -> Comparator/2
  Increment Decrement/1 -> ExtractBit/1, ExtractBit1/1
  GND/1 -> Increment Decrement/2
  n-to-1 Multiplexer/1 -> Angle[20:0]/1
  Pipelined Adder1/1 -> n-to-1 Multiplexer/2
  Degree90_1/1 -> Pipelined Adder1/2
  ExtractBit/1 -> n-to-1 Multiplexer/1
  Delay1/1 -> oNegAngle/1
  GND1/1 -> Delay1/3
  ExtractBit1/1 -> Delay1/1
  In1[20:0]/1 -> Comparator1/2, n-to-1 Multiplexer1/2, BusConversion/1
  Constant/1 -> Comparator1/1
  Comparator1/1 -> n-to-1 Multiplexer1/1
  n-to-1 Multiplexer1/1 -> Pipelined Adder/2
  BusConversion/1 -> n-to-1 Multiplexer1/3

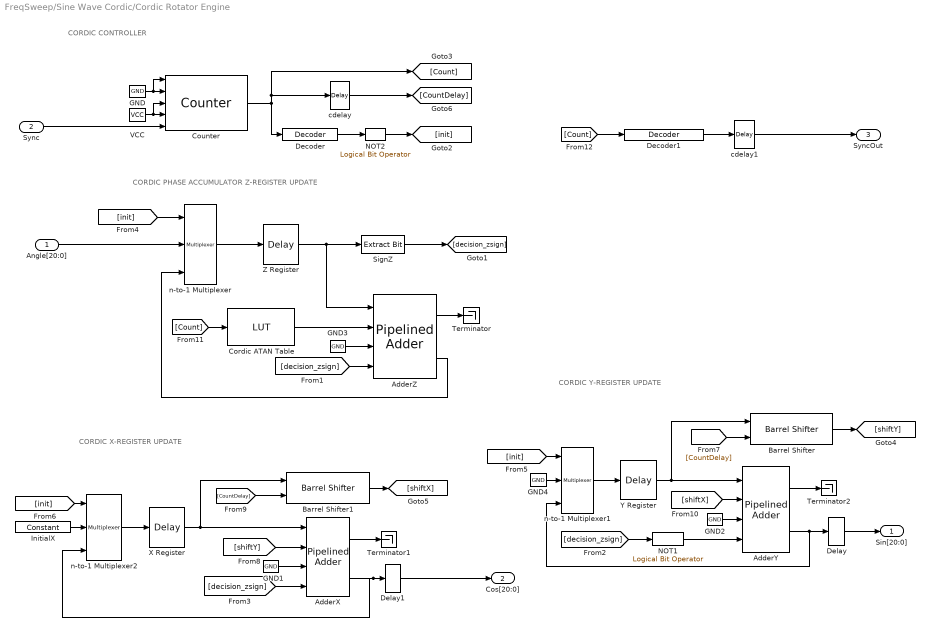
== system FreqSweep/Sine Wave Cordic/Cordic Rotator Engine ==
  note: CORDIC CONTROLLER
  note: CORDIC PHASE ACCUMULATOR Z-REGISTER UPDATE
  note: CORDIC X-REGISTER UPDATE
  note: CORDIC Y-REGISTER UPDATE
  Angle[20:0] : Inport
  Sync : Inport  Port=2
  AdderX : allblocks_alteradspbuilder2/Pipelined Adder  BusType=Signed Integer  bwl=21  bwr=0  pipeline=0  pipeline_display=0  AddSubDirection=ADD  use_cin=on  use_ovl=on  use_addsub=on  use_ena=on  use_aclr=on  or_aclr_inputs=on
  AdderY : allblocks_alteradspbuilder2/Pipelined Adder  BusType=Signed Integer  bwl=21  bwr=0  pipeline=0  pipeline_display=0  AddSubDirection=ADD  use_cin=on  use_ovl=on  use_addsub=on  use_ena=on  use_aclr=on  or_aclr_inputs=on
  AdderZ : allblocks_alteradspbuilder2/Pipelined Adder  BusType=Signed Integer  bwl=21  bwr=0  pipeline=0  pipeline_display=0  AddSubDirection=ADD  use_cin=on  use_ovl=on  use_addsub=on  use_ena=on  use_aclr=on  or_aclr_inputs=on
  Barrel Shifter : allblocks_alteradspbuilder2/Barrel Shifter  BusType=Signed Integer  bwl=21  bwr=0  pipeline=off  infer_distance=on  distance_length=8  ShiftDirection=Shift right  use_ena=off  use_aclr=off  UseDedicatedCircuitry=off  pipeline_display=0  allowFloatingPointOverride=on  logOutputs=off  logFile=/data/akarapet/qshell_linux64_test/p4/dsp_builder/dsp_builder2/Documentation/DesignExamples/Tutorials/HIL/FreqSweep/tb_FreqSweep/FreqSweep_Sine+Wave+Cordic_Cordic+Rotator+Engine_Barrel+Shifter.fixedpointlog
  Barrel Shifter1 : allblocks_alteradspbuilder2/Barrel Shifter  BusType=Signed Integer  bwl=21  bwr=0  pipeline=off  infer_distance=on  distance_length=8  ShiftDirection=Shift right  use_ena=off  use_aclr=off  UseDedicatedCircuitry=off  pipeline_display=0  allowFloatingPointOverride=on  logOutputs=off  logFile=/data/akarapet/qshell_linux64_test/p4/dsp_builder/dsp_builder2/Documentation/DesignExamples/Tutorials/HIL/FreqSweep/tb_FreqSweep/FreqSweep_Sine+Wave+Cordic_Cordic+Rotator+Engine_Barrel+Shifter1.fixedpointlog
  "Cordic ATAN Table " : allblocks_alteradspbuilder2/LUT  addr_width=5  BusType=Signed Integer  bwl=20  bwr=0  init_array=cordic_atan_table  allowFloatingPointOverride=on  logOutputs=off  logFile=/data/akarapet/qshell_linux64_test/p4/dsp_builder/dsp_builder2/Documentation/DesignExamples/Tutorials/HIL/FreqSweep/tb_FreqSweep/FreqSweep_Sine+Wave+Cordic_Cordic+Rotator+Engine_Cordic+ATAN+Table+.fixedpointlog  use_ena=off  reg_data=off  use_lpm=off  reg_addr=on  ram_type=AUTO  pipeline_display=1
  Counter : allblocks_alteradspbuilder2/Counter  BusType=Unsigned Integer  bwl=5  bwr=0  use_modulo=on  modulo=20  SpecifyClock=off  direction=Use Direction Port (updown)  use_sload=on  use_sset=off  svalue=1  use_clk_ena=off  use_ena=on  use_sclr=on  pipeline_display=1
  Decoder : allblocks_alteradspbuilder2/Decoder  BusType=Unsigned Integer  bwl=5  bwr=0  registered=off  pipeline_display=0  value=0
  Decoder1 : allblocks_alteradspbuilder2/Decoder  BusType=Unsigned Integer  bwl=5  bwr=0  registered=off  pipeline_display=0  value=19
  Delay : allblocks_alteradspbuilder2/Delay  pipeline=1  pipeline_display=1  ClockPhase=1  use_ena=off  use_sclr=off  allowFloatingPointOverride=on  logOutputs=off  logFile=/data/akarapet/qshell_linux64_test/p4/dsp_builder/dsp_builder2/Documentation/DesignExamples/Tutorials/HIL/FreqSweep/tb_FreqSweep/FreqSweep_Sine+Wave+Cordic_Cordic+Rotator+Engine_Delay.fixedpointlog  use_init=off  reset_value=1
  Delay1 : allblocks_alteradspbuilder2/Delay  pipeline=1  pipeline_display=1  ClockPhase=1  use_ena=off  use_sclr=off  allowFloatingPointOverride=on  logOutputs=off  logFile=/data/akarapet/qshell_linux64_test/p4/dsp_builder/dsp_builder2/Documentation/DesignExamples/Tutorials/HIL/FreqSweep/tb_FreqSweep/FreqSweep_Sine+Wave+Cordic_Cordic+Rotator+Engine_Delay1.fixedpointlog  use_init=off  reset_value=1
  GND{,1..4} (5 alike) : allblocks_alteradspbuilder2/GND  SpecifyClock=off
  InitialX : allblocks_alteradspbuilder2/Constant  mask_cst=round(0.60725293510314*ScalingFactor)  BusType=Signed Integer  bwl=20  bwr=0  roundMode=Truncate  satMode=Wrap  SpecifyClock=off  allowFloatingPointOverride=on  logOutputs=off  logFile=/data/akarapet/qshell_linux64_test/p4/dsp_builder/dsp_builder2/Documentation/DesignExamples/Tutorials/HIL/FreqSweep/tb_FreqSweep/FreqSweep_Sine+Wave+Cordic_Cordic+Rotator+Engine_InitialX.fixedpointlog
  NOT1 : allblocks_alteradspbuilder2/Logical Bit Operator  LogicalOperator=NOT  user_inputs=2  pipeline_display=0
  NOT2 : allblocks_alteradspbuilder2/Logical Bit Operator  LogicalOperator=NOT  user_inputs=2  pipeline_display=0
  SignZ : allblocks_alteradspbuilder2/Extract Bit  BusType=Signed Fractional  bwl=21  bwr=0  bitToSelect=20  pipeline_display=0
  Terminator : Terminator
  Terminator1 : Terminator
  Terminator2 : Terminator
  VCC : allblocks_alteradspbuilder2/VCC  SpecifyClock=off
  X Register : allblocks_alteradspbuilder2/Delay  pipeline=1  pipeline_display=1  ClockPhase=1  use_ena=off  use_sclr=off  allowFloatingPointOverride=on  logOutputs=off  logFile=/data/akarapet/qshell_linux64_test/p4/dsp_builder/dsp_builder2/Documentation/DesignExamples/Tutorials/HIL/FreqSweep/tb_FreqSweep/FreqSweep_Sine+Wave+Cordic_Cordic+Rotator+Engine_X+Register.fixedpointlog  use_init=off  reset_value=1
  Y Register : allblocks_alteradspbuilder2/Delay  pipeline=1  pipeline_display=1  ClockPhase=1  use_ena=off  use_sclr=off  allowFloatingPointOverride=on  logOutputs=off  logFile=/data/akarapet/qshell_linux64_test/p4/dsp_builder/dsp_builder2/Documentation/DesignExamples/Tutorials/HIL/FreqSweep/tb_FreqSweep/FreqSweep_Sine+Wave+Cordic_Cordic+Rotator+Engine_Y+Register.fixedpointlog  use_init=off  reset_value=1
  Z Register : allblocks_alteradspbuilder2/Delay  pipeline=1  pipeline_display=1  ClockPhase=1  use_ena=off  use_sclr=off  allowFloatingPointOverride=on  logOutputs=off  logFile=/data/akarapet/qshell_linux64_test/p4/dsp_builder/dsp_builder2/Documentation/DesignExamples/Tutorials/HIL/FreqSweep/tb_FreqSweep/FreqSweep_Sine+Wave+Cordic_Cordic+Rotator+Engine_Z+Register.fixedpointlog  use_init=off  reset_value=1
  cdelay : allblocks_alteradspbuilder2/Delay  pipeline=1  pipeline_display=1  ClockPhase=1  use_ena=off  use_sclr=off  allowFloatingPointOverride=on  logOutputs=off  logFile=/data/akarapet/qshell_linux64_test/p4/dsp_builder/dsp_builder2/Documentation/DesignExamples/Tutorials/HIL/FreqSweep/tb_FreqSweep/FreqSweep_Sine+Wave+Cordic_Cordic+Rotator+Engine_cdelay.fixedpointlog  use_init=off  reset_value=1
  cdelay1 : allblocks_alteradspbuilder2/Delay  pipeline=2  pipeline_display=2  ClockPhase=1  use_ena=off  use_sclr=off  allowFloatingPointOverride=on  logOutputs=off  logFile=/data/akarapet/qshell_linux64_test/p4/dsp_builder/dsp_builder2/Documentation/DesignExamples/Tutorials/HIL/FreqSweep/tb_FreqSweep/FreqSweep_Sine+Wave+Cordic_Cordic+Rotator+Engine_cdelay1.fixedpointlog  use_init=off  reset_value=1
  n-to-1 Multiplexer : allblocks_alteradspbuilder2/Multiplexer  numInputs=2  pipeline=0  oneHot=off  pipeline_display=0  use_ena=off  use_aclr=off  allowFloatingPointOverride=on  logOutputs=off  logFile=/data/akarapet/qshell_linux64_test/p4/dsp_builder/dsp_builder2/Documentation/DesignExamples/Tutorials/HIL/FreqSweep/tb_FreqSweep/FreqSweep_Sine+Wave+Cordic_Cordic+Rotator+Engine_n-to-1+Multiplexer.fixedpointlog
  n-to-1 Multiplexer1 : allblocks_alteradspbuilder2/Multiplexer  numInputs=2  pipeline=0  oneHot=off  pipeline_display=0  use_ena=off  use_aclr=off  allowFloatingPointOverride=on  logOutputs=off  logFile=/data/akarapet/qshell_linux64_test/p4/dsp_builder/dsp_builder2/Documentation/DesignExamples/Tutorials/HIL/FreqSweep/tb_FreqSweep/FreqSweep_Sine+Wave+Cordic_Cordic+Rotator+Engine_n-to-1+Multiplexer1.fixedpointlog
  n-to-1 Multiplexer2 : allblocks_alteradspbuilder2/Multiplexer  numInputs=2  pipeline=0  oneHot=off  pipeline_display=0  use_ena=off  use_aclr=off  allowFloatingPointOverride=on  logOutputs=off  logFile=/data/akarapet/qshell_linux64_test/p4/dsp_builder/dsp_builder2/Documentation/DesignExamples/Tutorials/HIL/FreqSweep/tb_FreqSweep/FreqSweep_Sine+Wave+Cordic_Cordic+Rotator+Engine_n-to-1+Multiplexer2.fixedpointlog
  Sin[20:0] : Outport
  Cos[20:0] : Outport  Port=2
  SyncOut : Outport  Port=3
  wires:
  Angle[20:0]/1 -> n-to-1 Multiplexer/2
  Sync/1 -> Counter/5
  GND/1 -> Counter/2, Counter/1
  VCC/1 -> Counter/4, Counter/3
  GND1/1 -> AdderX/3
  GND2/1 -> AdderY/3
  AdderX/2 -> n-to-1 Multiplexer2/3, Delay1/1
  AdderY/2 -> n-to-1 Multiplexer1/3, Delay/1
  Y Register/1 -> AdderY/1, Barrel Shifter/1
  X Register/1 -> AdderX/1, Barrel Shifter1/1
  n-to-1 Multiplexer/1 -> Z Register/1
  GND3/1 -> AdderZ/3
  Z Register/1 -> AdderZ/1, SignZ/1
  SignZ/1 -> [decision_zsign]
  [decision_zsign] -> AdderZ/4
  NOT1/1 -> AdderY/4
  [decision_zsign] -> NOT1/1
  Decoder/1 -> NOT2/1
  [init] -> n-to-1 Multiplexer/1
  [init] -> n-to-1 Multiplexer1/1
  n-to-1 Multiplexer1/1 -> Y Register/1
  GND4/1 -> n-to-1 Multiplexer1/2
  [decision_zsign] -> AdderX/4
  [init] -> n-to-1 Multiplexer2/1
  InitialX/1 -> n-to-1 Multiplexer2/2
  n-to-1 Multiplexer2/1 -> X Register/1
  [CountDelay] -> Barrel Shifter/2
  Barrel Shifter/1 -> [shiftY]
  [shiftY] -> AdderX/2
  [CountDelay] -> Barrel Shifter1/2
  Barrel Shifter1/1 -> [shiftX]
  [shiftX] -> AdderY/2
  "Cordic ATAN Table "/1 -> AdderZ/2
  [Count] -> "Cordic ATAN Table "/1
  Counter/1 -> Decoder/1, cdelay/1, [Count]
  AdderZ/2 -> n-to-1 Multiplexer/3
  NOT2/1 -> [init]
  cdelay/1 -> [CountDelay]
  Decoder1/1 -> cdelay1/1
  cdelay1/1 -> SyncOut/1
  [Count] -> Decoder1/1
  Delay/1 -> Sin[20:0]/1
  Delay1/1 -> Cos[20:0]/1
  AdderZ/1 -> Terminator/1
  AdderX/1 -> Terminator1/1
  AdderY/1 -> Terminator2/1

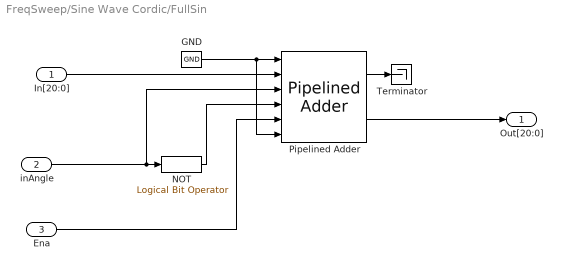
== system FreqSweep/Sine Wave Cordic/FullSin ==
  In[20:0] : Inport
  inAngle : Inport  Port=2
  Ena : Inport  Port=3
  GND : allblocks_alteradspbuilder2/GND  SpecifyClock=off
  NOT : allblocks_alteradspbuilder2/Logical Bit Operator  LogicalOperator=NOT  user_inputs=2  pipeline_display=0
  Pipelined Adder : allblocks_alteradspbuilder2/Pipelined Adder  BusType=Signed Integer  bwl=21  bwr=0  pipeline=2  pipeline_display=2  AddSubDirection=ADD  use_cin=on  use_ovl=on  use_addsub=on  use_ena=on  use_aclr=on  or_aclr_inputs=on
  Terminator : Terminator
  Out[20:0] : Outport
  wires:
  inAngle/1 -> NOT/1, Pipelined Adder/3
  In[20:0]/1 -> Pipelined Adder/2
  NOT/1 -> Pipelined Adder/4
  GND/1 -> Pipelined Adder/1, Pipelined Adder/6
  Pipelined Adder/2 -> Out[20:0]/1
  Ena/1 -> Pipelined Adder/5
  Pipelined Adder/1 -> Terminator/1
